simulink model "Second_Method"  (R2016b)
settings: Solver=VariableStepAuto  StartTime=0.0  StopTime=10.0  RelTol=1e-3
libraries: dspmtrx3 x1
settings Model: Creator=vbele  LastModifiedBy=vbele

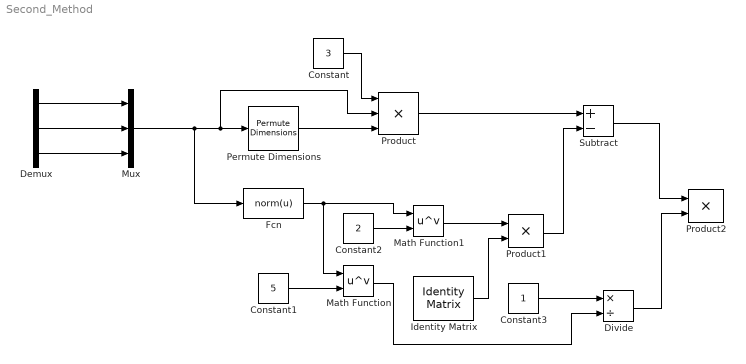
== system Second_Method ==
  Constant : Constant  Value=3
  Constant1 : Constant  Value=5
  Constant2 : Constant  Value=2
  Constant3 : Constant
  Demux : Demux  Outputs=3
  Divide : Product  Inputs=*/
  Fcn : Fcn  Expr=norm(u)
  Identity Matrix : dspmtrx3/Identity Matrix  Inherit=off  N=3  Ts=1  dataType=double  isSigned=on  wordLen=16  udDataType=sfix(16)  fracBitsMode=Best precision  numFracBits=15  OutDataTypeStr=double  LastOutDataTypeStr=double
  Math Function : Math  Operator=pow  SaturateOnIntegerOverflow=on
  Math Function1 : Math  Operator=pow  SaturateOnIntegerOverflow=on
  Mux : Mux  Inputs=3
  Permute Dimensions : PermuteDimensions
  Product : Product  Inputs=3
  Product1 : Product
  Product2 : Product
  Subtract : Sum  Inputs=+-
  wires:
  Demux/1 -> Mux/1
  Demux/2 -> Mux/2
  Demux/3 -> Mux/3
  Mux/1 -> Product/2, Permute Dimensions/1, Fcn/1
  Permute Dimensions/1 -> Product/3
  Constant/1 -> Product/1
  Fcn/1 -> Math Function/1, Math Function1/1
  Constant1/1 -> Math Function/2
  Constant2/1 -> Math Function1/2
  Identity Matrix/1 -> Product1/2
  Math Function1/1 -> Product1/1
  Product1/1 -> Subtract/2
  Product/1 -> Subtract/1
  Constant3/1 -> Divide/1
  Math Function/1 -> Divide/2
  Subtract/1 -> Product2/1
  Divide/1 -> Product2/2
